simulink model "process_ss"  (R2018b)
settings: Solver=FixedStepAuto  StartTime=0.0  StopTime=10000  FixedStep=1e-2  MaxStep=1  RelTol=1e-3
libraries: simulink x3
settings Model: Creator=smf52  LastModifiedBy=jh2044

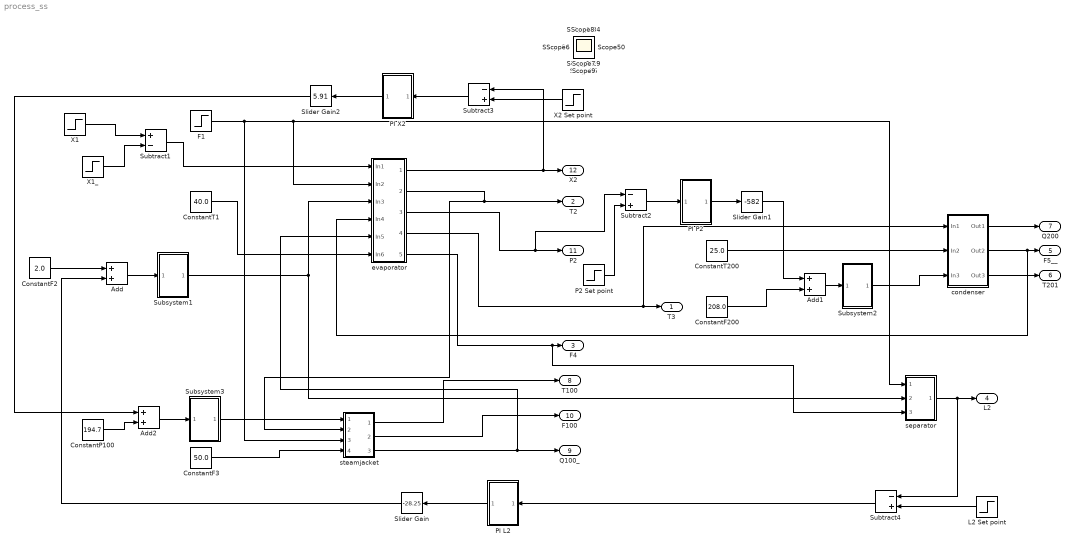
== system process_ss ==
  Add : Sum
  Add1 : Sum
  Add2 : Sum
  ConstantF2 : Constant  Value=2.0
  ConstantF200 : Constant  Value=208.0
  ConstantF3 : Constant  Value=50.0
  ConstantP100 : Constant  Value=194.7
  ConstantT1 : Constant  Value=40.0
  ConstantT200 : Constant  Value=25.0
  F1 : Step  Time=4000  Before=10  After=12  SampleTime=0
  L2 Set point : Step  Time=2000  Before=1  SampleTime=0
  P2 Set point : Step  Time=2000  Before=50.5  After=50.5  SampleTime=0
  PI L2 : Subsystem
  PI P2 : Subsystem
  PI X2 : Subsystem
  Slider Gain : simulink/Math Operations/Slider Gain  gain=-28.25  low=-100  high=0
  Slider Gain1 : simulink/Math Operations/Slider Gain  gain=-582  low=-1000  high=0
  Slider Gain2 : simulink/Math Operations/Slider Gain  gain=5.91  low=0  high=100
  Subsystem1 : Subsystem
  Subsystem2 : Subsystem
  Subsystem3 : Subsystem
  Subtract1 : Sum  Inputs=+-
  Subtract2 : Sum  Inputs=-+
  Subtract3 : Sum  Inputs=-+
  Subtract4 : Sum  Inputs=-+
  X1 : Step  Time=200  Before=5  After=25  SampleTime=0
  X1_ : Step  Time=300  After=0  SampleTime=0
  X2 Set point : Step  Time=2000  Before=25  After=25  SampleTime=0
  condenser : Subsystem
  evaporator : Subsystem
  separator : Subsystem
  steamjacket : Subsystem
  "T3 " : Outport
  T2 : Outport  Port=2
  F4 : Outport  Port=3
  "L2 " : Outport  Port=4
  F5__ : Outport  Port=5
  T201 : Outport  Port=6
  Q200 : Outport  Port=7
  T100 : Outport  Port=8
  Q100_ : Outport  Port=9
  F100 : Outport  Port=10
  "P2 " : Outport  Port=11
  X2 : Outport  Port=12
  Scope{,1..22} (23 alike) : Scope
  wires:
  condenser/2(Out2) -> evaporator/4(In4), F5__/1
  steamjacket/3(Out3) -> Q100_/1, evaporator/5(In5)
  ConstantT1/1 -> evaporator/6(In6)
  evaporator/1(Out1) -> Subtract3/1, X2/1
  evaporator/3(Out3) -> Subtract2/1, "P2 "/1
  F1/1 -> separator/1(In1), evaporator/2(In2), steamjacket/3(In3)
  evaporator/5(Out5) -> separator/3(In3), F4/1
  separator/1(Out1) -> Subtract4/1, "L2 "/1
  evaporator/2(Out2) -> T2/1, steamjacket/2(In2)
  ConstantF3/1 -> steamjacket/4(In4)
  steamjacket/1(Out1) -> T100/1
  steamjacket/2(Out2) -> F100/1
  evaporator/4(Out4) -> condenser/1(In1), "T3 "/1
  ConstantT200/1 -> condenser/2(In2)
  condenser/1(Out1) -> Q200/1
  condenser/3(Out3) -> T201/1
  ConstantF2/1 -> Add/1
  Slider Gain/1 -> Add/2
  Add/1 -> Subsystem1/1(In1)
  Subsystem1/1(Out1) -> separator/2(In2), evaporator/3(In3)
  Subsystem2/1(Out1) -> condenser/3(In3)
  Subsystem3/1(Out1) -> steamjacket/1(In1)
  PI L2/1(Out1) -> Slider Gain/1
  X1_/1 -> Subtract1/2
  X1/1 -> Subtract1/1
  Subtract1/1 -> evaporator/1(In1)
  P2 Set point/1 -> Subtract2/2
  Subtract2/1 -> PI P2/1(In1)
  PI P2/1(Out1) -> Slider Gain1/1
  Add1/1 -> Subsystem2/1(In1)
  Slider Gain1/1 -> Add1/1
  ConstantF200/1 -> Add1/2
  ConstantP100/1 -> Add2/2
  Add2/1 -> Subsystem3/1(In1)
  PI X2/1(Out1) -> Slider Gain2/1
  Subtract3/1 -> PI X2/1(In1)
  X2 Set point/1 -> Subtract3/2
  L2 Set point/1 -> Subtract4/2
  Subtract4/1 -> PI L2/1(In1)
  Slider Gain2/1 -> Add2/1

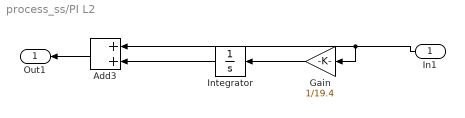
== system process_ss/PI L2 ==
  In1 : Inport
  Add3 : Sum
  Gain : Gain  Gain=1/19.4
  Integrator : Integrator
  Out1 : Outport
  wires:
  Gain/1 -> Integrator/1
  In1/1 -> Add3/1, Gain/1
  Add3/1 -> Out1/1
  Integrator/1 -> Add3/2

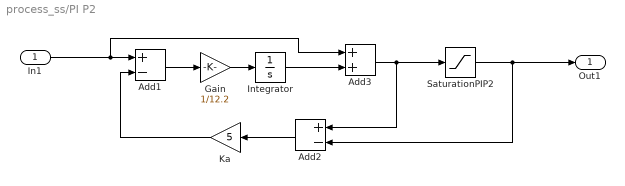
== system process_ss/PI P2 ==
  In1 : Inport
  Add1 : Sum  Inputs=+-
  Add2 : Sum  Inputs=+-
  Add3 : Sum
  Gain : Gain  Gain=1/12.2
  Integrator : Integrator
  Ka : Gain  Gain=5
  "SaturationPIP2 " : Saturate  LowerLimit=0
  Out1 : Outport
  wires:
  Gain/1 -> Integrator/1
  In1/1 -> Add1/1, Add3/1
  Integrator/1 -> Add3/2
  Add1/1 -> Gain/1
  "SaturationPIP2 "/1 -> Out1/1, Add2/2
  Add2/1 -> Ka/1
  Ka/1 -> Add1/2
  Add3/1 -> Add2/1, "SaturationPIP2 "/1

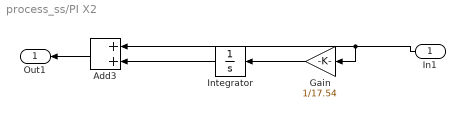
== system process_ss/PI X2 ==
  In1 : Inport
  Add3 : Sum
  Gain : Gain  Gain=1/17.54
  Integrator : Integrator
  Out1 : Outport
  wires:
  Gain/1 -> Integrator/1
  In1/1 -> Add3/1, Gain/1
  Add3/1 -> Out1/1
  Integrator/1 -> Add3/2

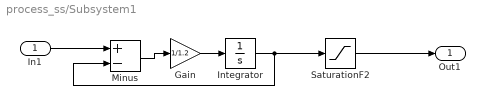
== system process_ss/Subsystem1 ==
  In1 : Inport
  Gain : Gain  Gain=1/1.2
  Integrator : Integrator  InitialCondition=2.0
  Minus : Sum  Inputs=+-
  "SaturationF2 " : Saturate  UpperLimit=4  LowerLimit=0
  Out1 : Outport
  wires:
  Gain/1 -> Integrator/1
  In1/1 -> Minus/1
  "SaturationF2 "/1 -> Out1/1
  Minus/1 -> Gain/1
  Integrator/1 -> "SaturationF2 "/1, Minus/2

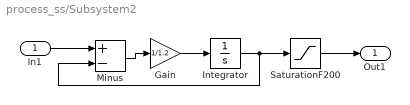
== system process_ss/Subsystem2 ==
  In1 : Inport
  Gain : Gain  Gain=1/1.2
  Integrator : Integrator  InitialCondition=208.0
  Minus : Sum  Inputs=+-
  "SaturationF200 " : Saturate  UpperLimit=416  LowerLimit=0
  Out1 : Outport
  wires:
  Gain/1 -> Integrator/1
  "SaturationF200 "/1 -> Out1/1
  In1/1 -> Minus/1
  Minus/1 -> Gain/1
  Integrator/1 -> "SaturationF200 "/1, Minus/2

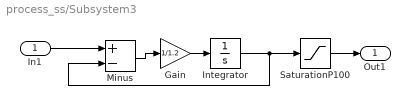
== system process_ss/Subsystem3 ==
  In1 : Inport
  Gain : Gain  Gain=1/1.2
  Integrator : Integrator  InitialCondition=194.7
  Minus : Sum  Inputs=+-
  "SaturationP100 " : Saturate  UpperLimit=400  LowerLimit=0
  Out1 : Outport
  wires:
  Gain/1 -> Integrator/1
  "SaturationP100 "/1 -> Out1/1
  In1/1 -> Minus/1
  Integrator/1 -> "SaturationP100 "/1, Minus/2
  Minus/1 -> Gain/1

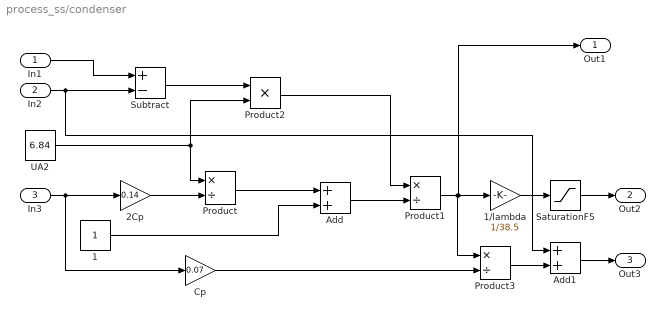
== system process_ss/condenser ==
  In1 : Inport
  In2 : Inport  Port=2
  In3 : Inport  Port=3
  1 : Constant
  1/lambda : Gain  Gain=1/38.5
  2Cp : Gain  Gain=0.14
  Add : Sum
  Add1 : Sum
  Cp : Gain  Gain=0.07
  Product : Product  Inputs=*/
  Product1 : Product  Inputs=*/
  Product2 : Product
  Product3 : Product  Inputs=*/
  "SaturationF5 " : Saturate  UpperLimit=16  LowerLimit=0
  Subtract : Sum  Inputs=+-
  UA2 : Constant  Value=6.84
  Out1 : Outport
  Out2 : Outport  Port=2
  Out3 : Outport  Port=3
  wires:
  Subtract/1 -> Product2/1
  1/1 -> Add/2
  Product2/1 -> Product1/1
  UA2/1 -> Product/1, Product2/2
  Add1/1 -> Out3/1
  In1/1 -> Subtract/1
  In2/1 -> Add1/1, Subtract/2
  Cp/1 -> Product3/2
  1/lambda/1 -> "SaturationF5 "/1
  In3/1 -> Cp/1, 2Cp/1
  Product3/1 -> Add1/2
  Add/1 -> Product1/2
  2Cp/1 -> Product/2
  Product1/1 -> Out1/1, 1/lambda/1, Product3/1
  Product/1 -> Add/1
  "SaturationF5 "/1 -> Out2/1

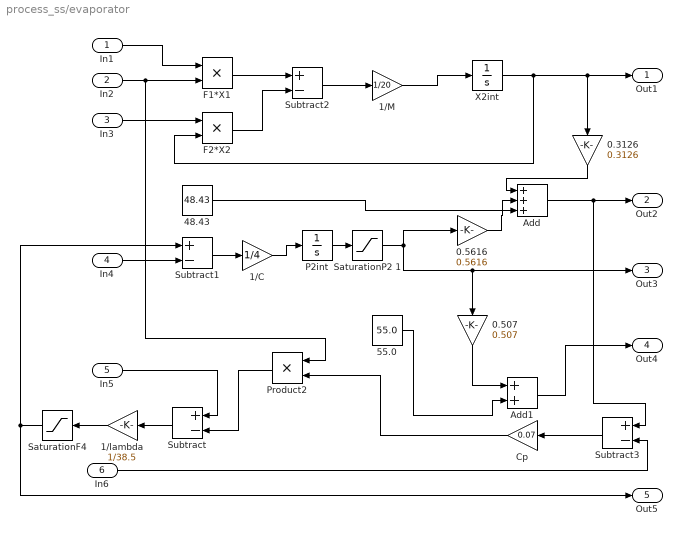
== system process_ss/evaporator ==
  In1 : Inport
  In2 : Inport  Port=2
  In3 : Inport  Port=3
  In4 : Inport  Port=4
  In5 : Inport  Port=5
  In6 : Inport  Port=6
  0.3126 : Gain  Gain=0.3126
  0.507 : Gain  Gain=0.507
  0.5616 : Gain  Gain=0.5616
  1/C : Gain  Gain=1/4
  1/M : Gain  Gain=1/20
  1/lambda : Gain  Gain=1/38.5
  48.43 : Constant  Value=48.43
  55.0 : Constant  Value=55.0
  Add : Sum  Inputs=+++
  Add1 : Sum
  Cp : Gain  Gain=0.07
  F1*X1 : Product
  F2*X2 : Product
  P2int : Integrator  InitialCondition=50.5
  Product2 : Product
  "SaturationF4 " : Saturate  UpperLimit=16  LowerLimit=0
  SaturationP2 1 : Saturate  UpperLimit=100  LowerLimit=0
  Subtract{,1..3} (4 alike) : Sum  Inputs=+-
  X2int : Integrator  InitialCondition=25
  Out1 : Outport
  Out2 : Outport  Port=2
  Out3 : Outport  Port=3
  Out4 : Outport  Port=4
  Out5 : Outport  Port=5
  wires:
  1/M/1 -> X2int/1
  F1*X1/1 -> Subtract2/1
  X2int/1 -> F2*X2/2, Out1/1, 0.3126/1
  55.0/1 -> Add1/2
  48.43/1 -> Add/3
  1/lambda/1 -> "SaturationF4 "/1
  In5/1 -> Subtract/1
  In2/1 -> Product2/1, F1*X1/2
  Subtract3/1 -> Cp/1
  In4/1 -> Subtract1/2
  Add1/1 -> Out4/1
  In1/1 -> F1*X1/1
  In6/1 -> Subtract3/2
  Subtract1/1 -> 1/C/1
  Product2/1 -> Subtract/2
  F2*X2/1 -> Subtract2/2
  Add/1 -> Out2/1, Subtract3/1
  Subtract2/1 -> 1/M/1
  Subtract/1 -> 1/lambda/1
  0.3126/1 -> Add/1
  0.5616/1 -> Add/2
  In3/1 -> F2*X2/1
  Cp/1 -> Product2/2
  0.507/1 -> Add1/1
  1/C/1 -> P2int/1
  "SaturationF4 "/1 -> Out5/1, Subtract1/1
  P2int/1 -> SaturationP2 1/1
  SaturationP2 1/1 -> Out3/1, 0.507/1, 0.5616/1

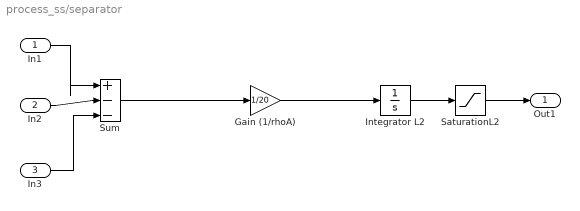
== system process_ss/separator ==
  In1 : Inport
  In2 : Inport  Port=2
  In3 : Inport  Port=3
  Gain (1/rhoA) : Gain  Gain=1/20
  "Integrator L2 " : Integrator  InitialCondition=1
  "SaturationL2 " : Saturate  UpperLimit=2  LowerLimit=0
  Sum : Sum  Inputs=|+--
  Out1 : Outport
  wires:
  In1/1 -> Sum/1
  Gain (1/rhoA)/1 -> "Integrator L2 "/1
  In3/1 -> Sum/3
  "Integrator L2 "/1 -> "SaturationL2 "/1
  Sum/1 -> Gain (1/rhoA)/1
  In2/1 -> Sum/2
  "SaturationL2 "/1 -> Out1/1

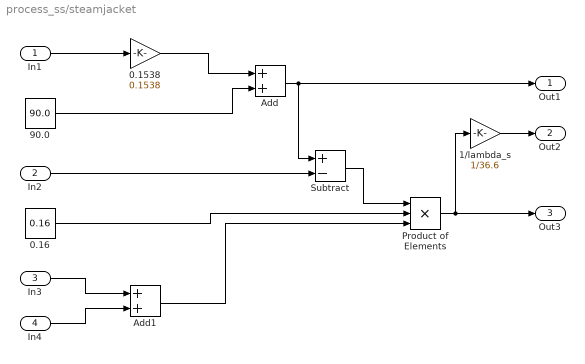
== system process_ss/steamjacket ==
  In1 : Inport
  In2 : Inport  Port=2
  In3 : Inport  Port=3
  In4 : Inport  Port=4
  0.1538 : Gain  Gain=0.1538
  0.16 : Constant  Value=0.16
  1/lambda_s : Gain  Gain=1/36.6
  90.0 : Constant  Value=90.0
  Add : Sum
  Add1 : Sum
  Product of Elements : Product  Inputs=***
  Subtract : Sum  Inputs=+-
  Out1 : Outport
  Out2 : Outport  Port=2
  Out3 : Outport  Port=3
  wires:
  In1/1 -> 0.1538/1
  0.16/1 -> Product of Elements/2
  In2/1 -> Subtract/2
  1/lambda_s/1 -> Out2/1
  Product of Elements/1 -> Out3/1, 1/lambda_s/1
  In4/1 -> Add1/2
  90.0/1 -> Add/2
  Subtract/1 -> Product of Elements/1
  0.1538/1 -> Add/1
  In3/1 -> Add1/1
  Add/1 -> Out1/1, Subtract/1
  Add1/1 -> Product of Elements/3
